simulink model "Subsystem"  (R2020b)
settings: Solver=FixedStepAuto  StartTime=0.0  StopTime=10.0  FixedStep=0.2  RelTol=1e-3
settings Model: Creator=Aradhana desai  LastModifiedBy=Aradhana desai
settings DataIOCC: SaveOutput=off  SaveTime=off

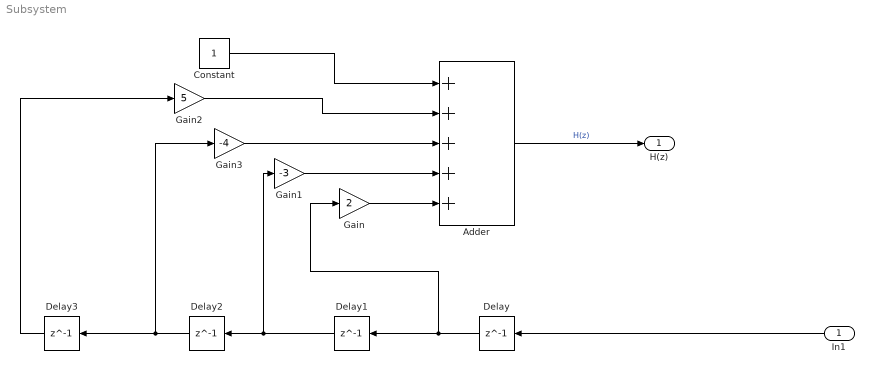
== system Subsystem ==
  In1 : Inport  OutDataTypeStr=double  PortDimensions=1  SampleTime=[0,1]
  Adder : Sum  Inputs=+++++
  Constant : Constant
  Delay{,1..3} (4 alike) : Delay  DelayLength=1
  Gain : Gain  Gain=2
  Gain1 : Gain  Gain=-3
  Gain2 : Gain  Gain=5
  Gain3 : Gain  Gain=-4
  H(z) : Outport  OutDataTypeStr=double  PortDimensions=1  SampleTime=[0.20000000000000001,0]
  wires:
  Gain/1 -> Adder/5
  Delay/1 -> Delay1/1, Gain/1
  Adder/1 -> H(z)/1  "H(z)"
  Gain3/1 -> Adder/3
  Delay1/1 -> Delay2/1, Gain1/1
  In1/1 -> Delay/1
  Delay3/1 -> Gain2/1
  Gain1/1 -> Adder/4
  Delay2/1 -> Delay3/1, Gain3/1
  Constant/1 -> Adder/1
  Gain2/1 -> Adder/2
